simulink model "Model"  (R2022a)
settings: Solver=VariableStepAuto  StartTime=0.0  StopTime=1  FixedStep=0.01  MaxStep=.01  RelTol=1e-3
values from neighbouring files (symbols this model uses):
  b = 3    [main.m]
  g = 9.81    [main.m]
  k = 0.9    [main.m]
  l = 0.5    [main.m]
  m = 1    [main.m]
undefined symbols (not defined in the file or in its folder): A, B, C, D, Regulator_AutoTune
settings Model: Creator=Pett  LastModifiedBy=Pett

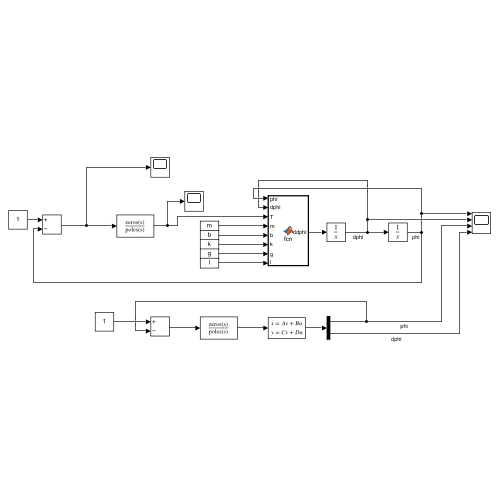
[thumbnail: Simulink's stored preview of the top-level diagram]
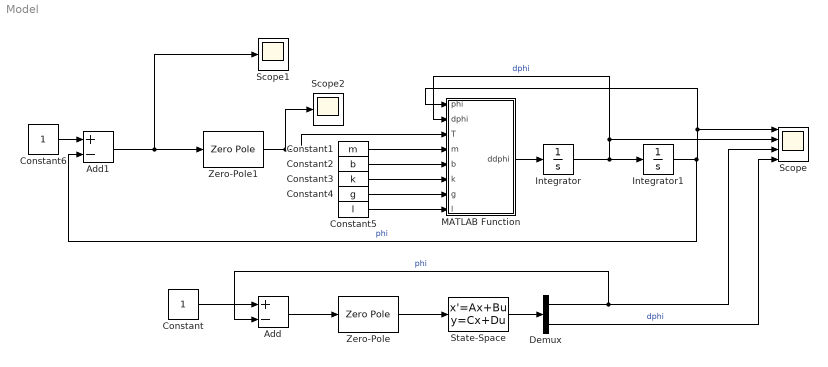
== system Model ==
  Add : Sum  Inputs=+-
  Add1 : Sum  Inputs=+-
  Constant : Constant
  Constant1 : Constant  Value=m
  Constant2 : Constant  Value=b
  Constant3 : Constant  Value=k
  Constant4 : Constant  Value=g
  Constant5 : Constant  Value=l
  Constant6 : Constant
  Demux : Demux  Outputs=2
  Integrator : Integrator
  Integrator1 : Integrator
  MATLAB Function : MATLAB Function  TreatAsAtomicUnit=on
  Scope : Scope  NumInputPorts=4
  Scope1 : Scope
  Scope2 : Scope
  State-Space : StateSpace  A=A  B=B  C=C  D=D  InitialCondition=0
  Zero-Pole : ZeroPole  Zeros=cell2mat(Regulator_AutoTune.Z)  Poles=cell2mat(Regulator_AutoTune.P)  Gain=Regulator_AutoTune.K
  Zero-Pole1 : ZeroPole  Zeros=cell2mat(Regulator_AutoTune.Z)  Poles=cell2mat(Regulator_AutoTune.P)  Gain=Regulator_AutoTune.K
  wires:
  Integrator/1 -> MATLAB Function/2(dphi), Scope/2, Integrator1/1  "dphi"
  Integrator1/1 -> Add1/2, MATLAB Function/1(phi), Scope/1  "phi"
  MATLAB Function/1(ddphi) -> Integrator/1
  Constant3/1 -> MATLAB Function/6(k)
  Constant1/1 -> MATLAB Function/4(m)
  Constant2/1 -> MATLAB Function/5(b)
  Constant4/1 -> MATLAB Function/7(g)
  Constant5/1 -> MATLAB Function/8(l)
  Constant/1 -> Add/1
  Add/1 -> Zero-Pole/1
  State-Space/1 -> Demux/1
  Demux/1 -> Add/2, Scope/3  "phi"
  Demux/2 -> Scope/4  "dphi"
  Zero-Pole1/1 -> Scope2/1, MATLAB Function/3(T)
  Constant6/1 -> Add1/1
  Add1/1 -> Scope1/1, Zero-Pole1/1
  Zero-Pole/1 -> State-Space/1

== matlab function Model/MATLAB Function ==
  data: phi input; ddphi output; dphi input; T input; m input; b input; k input; g input; l input
function ddphi = fcn(phi, dphi, T, m, b, k, g, l)

ddphi = -(b*dphi - T + k* phi + g*l*m*sin(phi))/(l^2*m);
